simulink model "AMR_ManualModeController_23b"  (R2023b)
settings: Solver=FixedStepAuto  StartTime=0.0  StopTime=inf  FixedStep=1e-3  RelTol=1e-3
model workspace (MAT data in the model file):
  mdlWSDbList = "C:\Users\matlab.cut\Desktop\AMR\canbus_files\tramontina_database_mobotic.dbc"
  mobotic_mechanical_offset = -30
libraries: hdlsllib x4, speedgoatlib_IO60X_IO69X x3, tramontina_database_moboticlib x3, slrealtimeutilitieslib x1
settings Model: Creator=matlab.cut  LastModifiedBy=matlab.cut
settings SolverCC: ConcurrentTasks=on  PositivePriorityOrder=on  AutoInsertRateTranBlk=on
settings OptimizationCC: BlockReduction=off  OptimizeBlockIOStorage=off
settings DebuggingCC: TasksWithSamePriorityMsg=none
settings HardwareCC: ProdBitPerLong=64  ProdLongLongMode=on  ProdHWDeviceType=Intel->x86-64 (Linux 64)
settings ModelReferenceCC: ModelReferenceNumInstancesAllowed=Single
settings RTWCC: Description=Simulink Real-Time  SystemTargetFile=slrealtime.tlc  TemplateMakefile=slrealtime_default_tmf  Toolchain=Simulink Real-Time Toolchain  BuildConfiguration=Faster Runs  CodeExecutionProfiling=on  TargetLang=C++
settings CodeAppCC: MaxIdLength=127

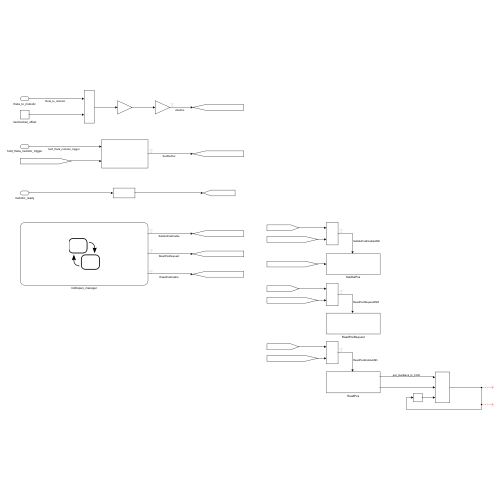
[thumbnail: Simulink's stored preview of the top-level diagram]
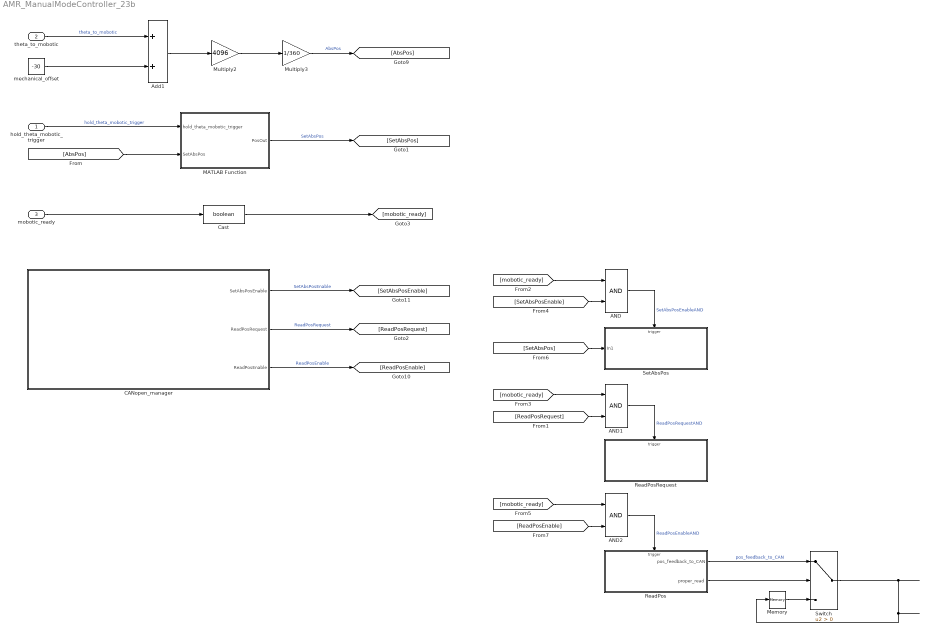
== system AMR_ManualModeController_23b ==
  hold_theta_mobotic_trigger : Inport  OutDataTypeStr=boolean
  theta_to_mobotic : Inport  Port=2
  mobotic_ready : Inport  Port=3  OutDataTypeStr=boolean
  AND : Logic  AllPortsSameDT=off  OutDataTypeStr=boolean
  AND1 : Logic  AllPortsSameDT=off  OutDataTypeStr=boolean
  AND2 : Logic  AllPortsSameDT=off  OutDataTypeStr=boolean
  Add1 : Sum
  CANopen_manager : Stateflow chart  TreatAsAtomicUnit=on
  Cast : DataTypeConversion  OutDataTypeStr=boolean  SaturateOnIntegerOverflow=off  RndMeth=Floor
  MATLAB Function : MATLAB Function  TreatAsAtomicUnit=on
  Memory : Memory
  Multiply2 : Gain  Gain=4096
  Multiply3 : Gain  Gain=1/360
  ReadPos : Subsystem  TreatAsAtomicUnit=on
  ReadPosRequest : Subsystem  TreatAsAtomicUnit=on
  SetAbsPos : Subsystem  TreatAsAtomicUnit=on
  Switch : Switch  Criteria=u2 > Threshold  SaturateOnIntegerOverflow=off  InputSameDT=off
  mechanical_offset : Constant  Value=-30
  wires:
  Multiply3/1 -> [AbsPos]  "AbsPos"
  CANopen_manager/3(ReadPosEnable) -> [ReadPosEnable]  "ReadPosEnable"
  mechanical_offset/1 -> Add1/2
  Add1/1 -> Multiply2/1
  [SetAbsPos] -> SetAbsPos/1(In1)
  Multiply2/1 -> Multiply3/1
  CANopen_manager/1(SetAbsPosEnable) -> [SetAbsPosEnable]  "SetAbsPosEnable"
  theta_to_mobotic/1 -> Add1/1  "theta_to_mobotic"
  [AbsPos] -> MATLAB Function/2(SetAbsPos)
  MATLAB Function/1(PosOut) -> [SetAbsPos]  "SetAbsPos"
  hold_theta_mobotic_trigger/1 -> MATLAB Function/1(hold_theta_mobotic_trigger)  "hold_theta_mobotic_trigger"
  CANopen_manager/2(ReadPosRequest) -> [ReadPosRequest]  "ReadPosRequest"
  ReadPos/2(proper_read) -> Switch/2
  Memory/1 -> Switch/3
  ReadPos/1(pos_feedback_to_CAN) -> Switch/1  "pos_feedback_to_CAN"
  Switch/1 -> Memory/1
  mobotic_ready/1 -> Cast/1
  AND/1 -> SetAbsPos/Trigger  "SetAbsPosEnableAND"
  [SetAbsPosEnable] -> AND/2
  [mobotic_ready] -> AND/1
  [mobotic_ready] -> AND1/1
  AND1/1 -> ReadPosRequest/Trigger  "ReadPosRequestAND"
  [ReadPosRequest] -> AND1/2
  [mobotic_ready] -> AND2/1
  [ReadPosEnable] -> AND2/2
  AND2/1 -> ReadPos/Trigger  "ReadPosEnableAND"
  Cast/1 -> [mobotic_ready]

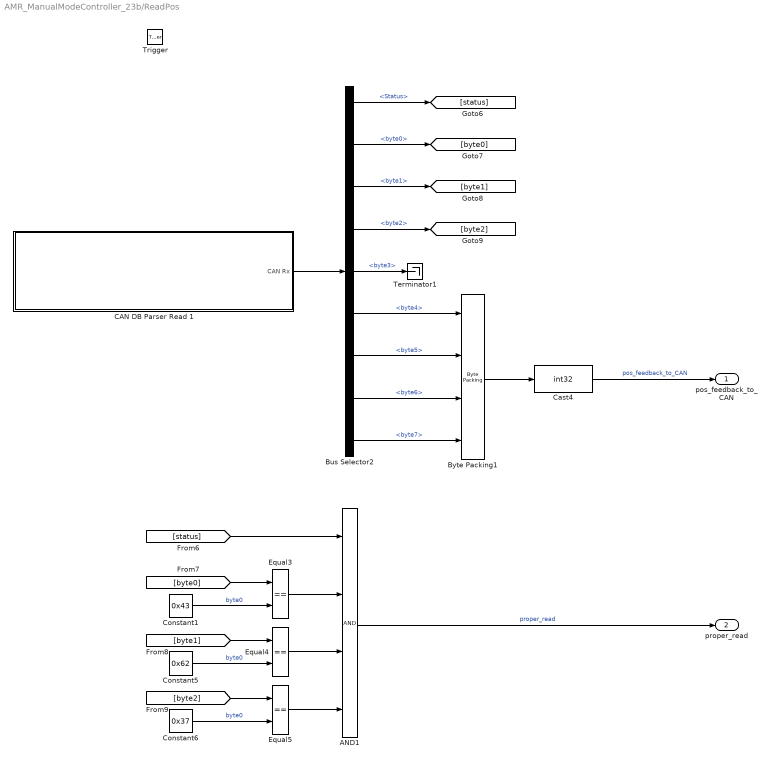
== system AMR_ManualModeController_23b/ReadPos ==
  Trigger : TriggerPort  VariantControl=(inherit)  PortDimensions=1
  AND1 : Logic  Inputs=4  AllPortsSameDT=off  OutDataTypeStr=boolean
  Bus Selector2 : BusSelector  OutputSignals=ID1459_feedback_word.MessageStatus.Status,ID1459_feedback_word.byte0,ID1459_feedback_word.byte1,ID1459_feedback_word.byte2,ID1459_feedback_word.byte3,ID1459_feedback_word.byte4,ID1459_feedback_word.byte5,ID1459_feedback_word.byte6,ID1459_feedback_word.byte7
  Byte Packing1 : slrealtimeutilitieslib/Byte Packing  MaskPackedDataType=int32  MaskUnpackedDataTypes={'uint8','uint8','uint8','uint8'}  MaskAlignment=1
  CAN DB Parser Read 1 : Subsystem
      settings: OpenFcn=sg_can.OpenFcnRead;
      mask Help: eval('sg.utils.help.show(''io_main/refentry_ref_can_ofa_parsing_read'');')
      mask Display: disp('Speedgoat\nIO691\nCAN DB Parser Read\nModule ID: IO691 - Module ID 1\nChannel:  1\ntramontina_database_mobotic.dbc ');
  Cast4 : DataTypeConversion  OutDataTypeStr=int32  SaturateOnIntegerOverflow=off  RndMeth=Floor
  Constant1 : Constant  Value=0x43
  Constant5 : Constant  Value=0x62
  Constant6 : Constant  Value=0x37
  Equal3 : RelationalOperator  Operator===  OutDataTypeStr=boolean  RndMeth=Simplest  InputSameDT=off
  Equal4 : RelationalOperator  Operator===  OutDataTypeStr=boolean  RndMeth=Simplest  InputSameDT=off
  Equal5 : RelationalOperator  Operator===  OutDataTypeStr=boolean  RndMeth=Simplest  InputSameDT=off
  Terminator1 : Terminator
  pos_feedback_to_CAN : Outport
  proper_read : Outport  Port=2
  wires:
  Equal5/1 -> AND1/4
  [byte0] -> Equal3/1
  Constant5/1 -> Equal4/2  "byte0"
  Bus Selector2/5 -> Terminator1/1  "<byte3>"
  [byte1] -> Equal4/1
  [byte2] -> Equal5/1
  Bus Selector2/9 -> Byte Packing1/4  "<byte7>"
  Bus Selector2/4 -> [byte2]  "<byte2>"
  [status] -> AND1/1
  Bus Selector2/2 -> [byte0]  "<byte0>"
  Bus Selector2/1 -> [status]  "<Status>"
  Bus Selector2/8 -> Byte Packing1/3  "<byte6>"
  Equal4/1 -> AND1/3
  AND1/1 -> proper_read/1  "proper_read"
  Bus Selector2/7 -> Byte Packing1/2  "<byte5>"
  Equal3/1 -> AND1/2
  Byte Packing1/1 -> Cast4/1
  CAN DB Parser Read 1/1(CAN Rx) -> Bus Selector2/1
  Bus Selector2/6 -> Byte Packing1/1  "<byte4>"
  Constant6/1 -> Equal5/2  "byte0"
  Bus Selector2/3 -> [byte1]  "<byte1>"
  Constant1/1 -> Equal3/2  "byte0"
  Cast4/1 -> pos_feedback_to_CAN/1  "pos_feedback_to_CAN"

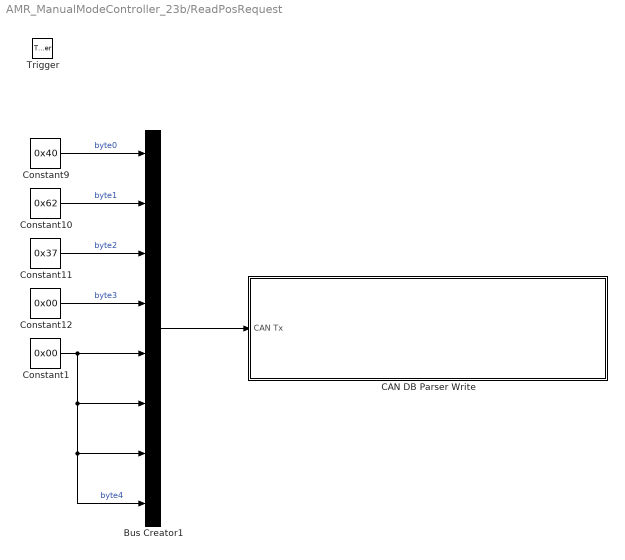
== system AMR_ManualModeController_23b/ReadPosRequest ==
  Trigger : TriggerPort  VariantControl=(inherit)  PortDimensions=1
  Bus Creator1 : BusCreator  Inputs=8
  "CAN DB Parser Write " : Subsystem
      settings: OpenFcn=sg_can.OpenFcnWrite;
      mask Help: eval('sg.utils.help.show(''io_main/refentry_ref_can_ofa_parsing_write'');')
      mask Display: disp('Speedgoat\nIO691\nCAN DB Parser Write\nModule ID: IO691 - Module ID 1\nChannel:  1\ntramontina_database_mobotic.dbc ');
  Constant1 : Constant  Value=0x00
  Constant10 : Constant  Value=0x62
  Constant11 : Constant  Value=0x37
  Constant12 : Constant  Value=0x00
  Constant9 : Constant  Value=0x40
  wires:
  Constant12/1 -> Bus Creator1/4  "byte3"
  Bus Creator1/1 -> "CAN DB Parser Write "/1(CAN Tx)
  Constant1/1 -> Bus Creator1/8, Bus Creator1/7, Bus Creator1/6, Bus Creator1/5  "byte4"
  Constant10/1 -> Bus Creator1/2  "byte1"
  Constant11/1 -> Bus Creator1/3  "byte2"
  Constant9/1 -> Bus Creator1/1  "byte0"

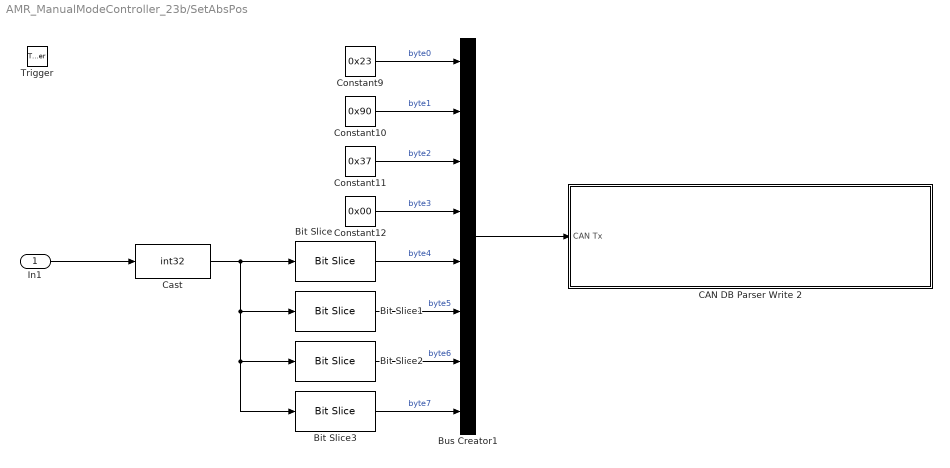
== system AMR_ManualModeController_23b/SetAbsPos ==
  In1 : Inport
  Trigger : TriggerPort  VariantControl=(inherit)  PortDimensions=1
  Bit Slice : hdlsllib/Logic and Bit Operations/Bit Slice  lidx=7  ridx=0
  Bit Slice1 : hdlsllib/Logic and Bit Operations/Bit Slice  lidx=15  ridx=8
  Bit Slice2 : hdlsllib/Logic and Bit Operations/Bit Slice  lidx=23  ridx=16
  Bit Slice3 : hdlsllib/Logic and Bit Operations/Bit Slice  lidx=31  ridx=24
  Bus Creator1 : BusCreator  Inputs=8
  CAN DB Parser Write 2 : Subsystem
      settings: OpenFcn=sg_can.OpenFcnWrite;
      mask Help: eval('sg.utils.help.show(''io_main/refentry_ref_can_ofa_parsing_write'');')
      mask Display: disp('Speedgoat\nIO691\nCAN DB Parser Write\nModule ID: IO691 - Module ID 1\nChannel:  1\ntramontina_database_mobotic.dbc ');
  Cast : DataTypeConversion  OutDataTypeStr=int32  SaturateOnIntegerOverflow=off  RndMeth=Floor
  Constant10 : Constant  Value=0x90
  Constant11 : Constant  Value=0x37
  Constant12 : Constant  Value=0x00
  Constant9 : Constant  Value=0x23
  wires:
  Constant9/1 -> Bus Creator1/1  "byte0"
  Constant12/1 -> Bus Creator1/4  "byte3"
  Constant11/1 -> Bus Creator1/3  "byte2"
  Bus Creator1/1 -> CAN DB Parser Write 2/1(CAN Tx)
  Constant10/1 -> Bus Creator1/2  "byte1"
  Bit Slice/1 -> Bus Creator1/5  "byte4"
  Bit Slice1/1 -> Bus Creator1/6  "byte5"
  Bit Slice2/1 -> Bus Creator1/7  "byte6"
  Bit Slice3/1 -> Bus Creator1/8  "byte7"
  In1/1 -> Cast/1
  Cast/1 -> Bit Slice3/1, Bit Slice2/1, Bit Slice1/1, Bit Slice/1

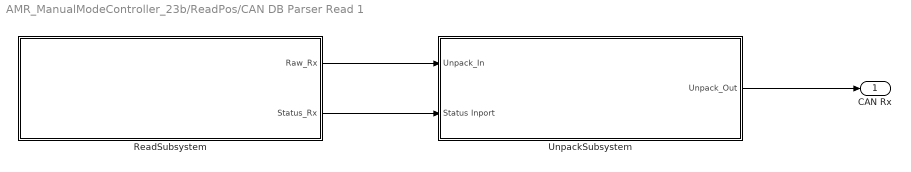
== system AMR_ManualModeController_23b/ReadPos/CAN DB Parser Read 1 ==
  ReadSubsystem : Subsystem
  UnpackSubsystem : Subsystem
  CAN Rx : Outport
  wires:
  ReadSubsystem/1(Raw_Rx) -> UnpackSubsystem/1(Unpack_In)
  ReadSubsystem/2(Status_Rx) -> UnpackSubsystem/2(Status Inport)
  UnpackSubsystem/1(Unpack_Out) -> CAN Rx/1

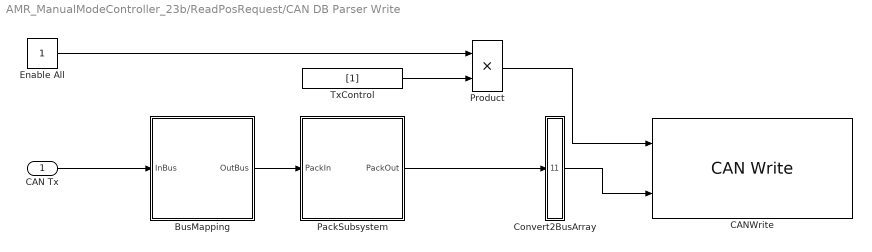
== system AMR_ManualModeController_23b/ReadPosRequest/CAN DB Parser Write  ==
  CAN Tx : Inport
  BusMapping : Subsystem
  CANWrite : speedgoatlib_IO60X_IO69X/CAN/CAN Write   moduleType=IO691  id=1  channel=1  canType=CAN (HS)  messageType=CAN (HS)  useBusIn=on  numOfMsg=1  enableInput=on  enableStatusPort=off  ts=-1  initValues=[691 1 -1 0 1 1 0 1 1 1]
  Convert2BusArray : Subsystem
  Enable All : Constant  OutDataTypeStr=boolean
  PackSubsystem : Subsystem
  Product : Product  OutDataTypeStr=uint32
  TxControl : Constant  Value=[1]  OutDataTypeStr=uint32
  wires:
  PackSubsystem/1(PackOut) -> Convert2BusArray/1(InBus)
  Convert2BusArray/1(BusArrayOut) -> CANWrite/2
  Product/1 -> CANWrite/1
  TxControl/1 -> Product/2
  Enable All/1 -> Product/1
  CAN Tx/1 -> BusMapping/1(InBus)
  BusMapping/1(OutBus) -> PackSubsystem/1(PackIn)

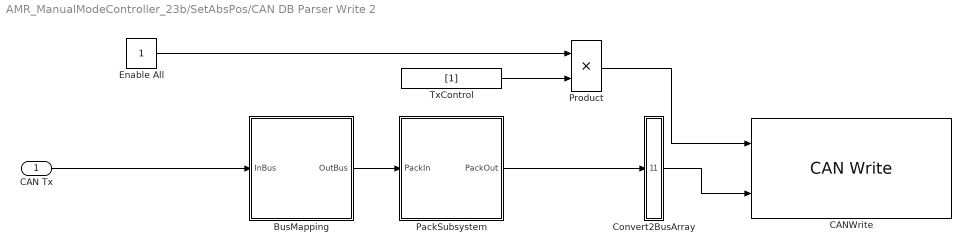
== system AMR_ManualModeController_23b/SetAbsPos/CAN DB Parser Write 2 ==
  CAN Tx : Inport
  BusMapping : Subsystem
  CANWrite : speedgoatlib_IO60X_IO69X/CAN/CAN Write   moduleType=IO691  id=1  channel=1  canType=CAN (HS)  messageType=CAN (HS)  useBusIn=on  numOfMsg=1  enableInput=on  enableStatusPort=off  ts=-1  initValues=[691 1 -1 0 1 1 0 1 1 1]
  Convert2BusArray : Subsystem
  Enable All : Constant  OutDataTypeStr=boolean
  PackSubsystem : Subsystem
  Product : Product  OutDataTypeStr=uint32
  TxControl : Constant  Value=[1]  OutDataTypeStr=uint32
  wires:
  PackSubsystem/1(PackOut) -> Convert2BusArray/1(InBus)
  Convert2BusArray/1(BusArrayOut) -> CANWrite/2
  Product/1 -> CANWrite/1
  TxControl/1 -> Product/2
  Enable All/1 -> Product/1
  CAN Tx/1 -> BusMapping/1(InBus)
  BusMapping/1(OutBus) -> PackSubsystem/1(PackIn)

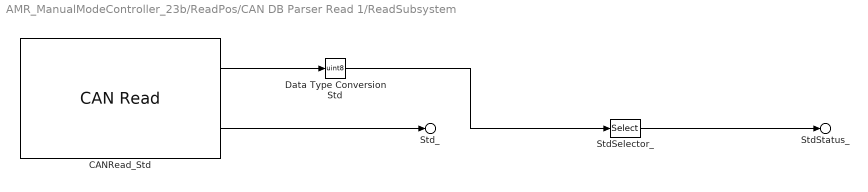
== system AMR_ManualModeController_23b/ReadPos/CAN DB Parser Read 1/ReadSubsystem ==
  CANRead_Std : speedgoatlib_IO60X_IO69X/CAN/CAN Read   moduleType=IO691  id=1  channel=1  canType=CAN (HS)  messageType=CAN (HS)  useBusOut=on  HasMulRead=Specify by IDs  MsgIDlist=[1459]  isEFF=off  LabelInHex=off  enableInput=off  initValues=[691 1 -1 0 1 1 0 1 2 0 1 1459]  ts=-1
  Data Type ConversionStd : DataTypeConversion  OutDataTypeStr=uint8  SaturateOnIntegerOverflow=off  RndMeth=Floor
  StdSelector_ : Selector  IndexOptions=Index vector (dialog)  Indices=1  OutputSizes=1
  Std_ : Outport  PortName=Raw_Rx  Element=Std.ID1459
  StdStatus_ : Outport  Port=2  PortName=Status_Rx  Element=Std.ID1459
  wires:
  CANRead_Std/1 -> Data Type ConversionStd/1
  CANRead_Std/2 -> Std_/1
  Data Type ConversionStd/1 -> StdSelector_/1
  StdSelector_/1 -> StdStatus_/1

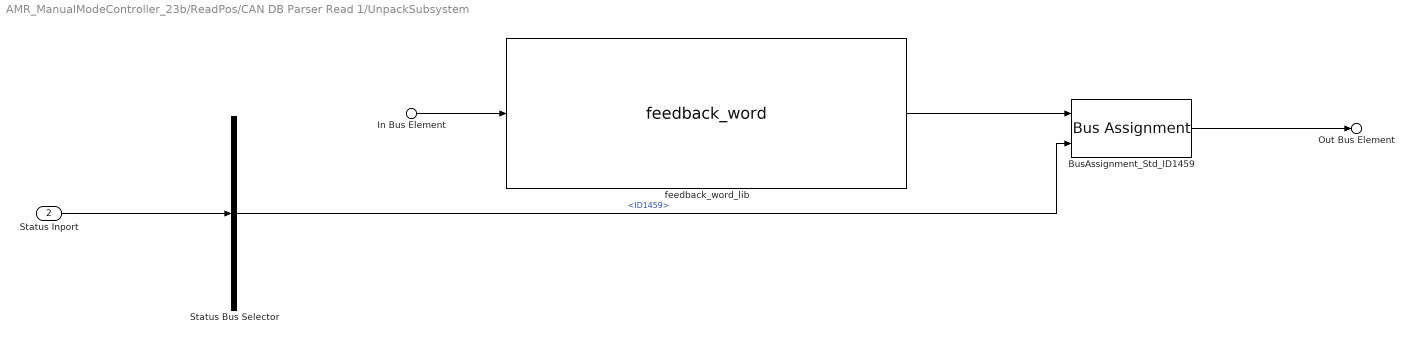
== system AMR_ManualModeController_23b/ReadPos/CAN DB Parser Read 1/UnpackSubsystem ==
  In Bus Element : Inport  PortName=Unpack_In  Element=Std.ID1459
  Status Inport : Inport  Port=2
  BusAssignment_Std_ID1459 : BusAssignment  AssignedSignals=MessageStatus.Status
  Status Bus Selector : BusSelector  OutputSignals=Std.ID1459
  feedback_word_lib : tramontina_database_moboticlib/CAN unpack/feedback_word  SystemSampleTime=-1  VariantActivationTime=update diagram  AllowFlexibleInterface=on  Latency=0  AutoFrameSizeCalculation=off
  Out Bus Element : Outport  PortName=Unpack_Out  Element=ID1459_feedback_word
  wires:
  In Bus Element/1 -> feedback_word_lib/1
  feedback_word_lib/1 -> BusAssignment_Std_ID1459/1
  BusAssignment_Std_ID1459/1 -> Out Bus Element/1
  Status Inport/1 -> Status Bus Selector/1
  Status Bus Selector/1 -> BusAssignment_Std_ID1459/2  "<ID1459>"

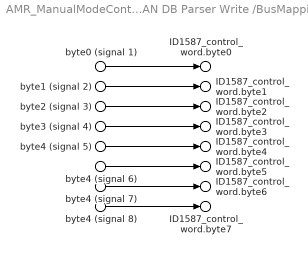
== system AMR_ManualModeController_23b/ReadPosRequest/CAN DB Parser Write /BusMapping ==
  byte0 (signal 1) : Inport  PortName=InBus  Element=byte0 (signal 1)
  byte1 (signal 2) : Inport  PortName=InBus  Element=byte1 (signal 2)
  byte2 (signal 3) : Inport  PortName=InBus  Element=byte2 (signal 3)
  byte3 (signal 4) : Inport  PortName=InBus  Element=byte3 (signal 4)
  byte4 (signal 5) : Inport  PortName=InBus  Element=byte4 (signal 5)
  byte4 (signal 6) : Inport  PortName=InBus  Element=byte4 (signal 6)
  byte4 (signal 7) : Inport  PortName=InBus  Element=byte4 (signal 7)
  byte4 (signal 8) : Inport  PortName=InBus  Element=byte4 (signal 8)
  ID1587_control_word.byte0 : Outport  PortName=OutBus  Element=ID1587_control_word.byte0
  ID1587_control_word.byte1 : Outport  PortName=OutBus  Element=ID1587_control_word.byte1
  ID1587_control_word.byte2 : Outport  PortName=OutBus  Element=ID1587_control_word.byte2
  ID1587_control_word.byte3 : Outport  PortName=OutBus  Element=ID1587_control_word.byte3
  ID1587_control_word.byte4 : Outport  PortName=OutBus  Element=ID1587_control_word.byte4
  ID1587_control_word.byte5 : Outport  PortName=OutBus  Element=ID1587_control_word.byte5
  ID1587_control_word.byte6 : Outport  PortName=OutBus  Element=ID1587_control_word.byte6
  ID1587_control_word.byte7 : Outport  PortName=OutBus  Element=ID1587_control_word.byte7
  wires:
  byte0 (signal 1)/1 -> ID1587_control_word.byte0/1
  byte1 (signal 2)/1 -> ID1587_control_word.byte1/1
  byte2 (signal 3)/1 -> ID1587_control_word.byte2/1
  byte3 (signal 4)/1 -> ID1587_control_word.byte3/1
  byte4 (signal 5)/1 -> ID1587_control_word.byte4/1
  byte4 (signal 6)/1 -> ID1587_control_word.byte5/1
  byte4 (signal 7)/1 -> ID1587_control_word.byte6/1
  byte4 (signal 8)/1 -> ID1587_control_word.byte7/1

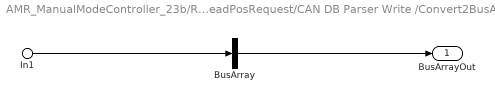
== system AMR_ManualModeController_23b/ReadPosRequest/CAN DB Parser Write /Convert2BusArray ==
  In1 : Inport  PortName=InBus  Element=ID1587_control_word
  BusArray : Concatenate  NumInputs=1
  BusArrayOut : Outport
  wires:
  In1/1 -> BusArray/1
  BusArray/1 -> BusArrayOut/1

== system AMR_ManualModeController_23b/ReadPosRequest/CAN DB Parser Write /PackSubsystem ==
  In Bus Element : Inport  PortName=PackIn  Element=ID1587_control_word
  control_word_lib : tramontina_database_moboticlib/CAN pack/control_word  SystemSampleTime=-1  VariantActivationTime=update diagram  AllowFlexibleInterface=on  Latency=0  AutoFrameSizeCalculation=off
  In Bus Element1 : Outport  PortName=PackOut  Element=ID1587_control_word
  wires:
  In Bus Element/1 -> control_word_lib/1
  control_word_lib/1 -> In Bus Element1/1

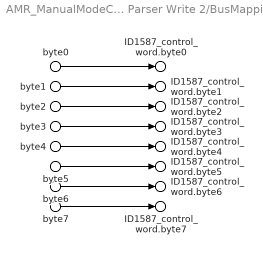
== system AMR_ManualModeController_23b/SetAbsPos/CAN DB Parser Write 2/BusMapping ==
  byte0 : Inport  PortName=InBus  Element=byte0
  byte1 : Inport  PortName=InBus  Element=byte1
  byte2 : Inport  PortName=InBus  Element=byte2
  byte3 : Inport  PortName=InBus  Element=byte3
  byte4 : Inport  PortName=InBus  Element=byte4
  byte5 : Inport  PortName=InBus  Element=byte5
  byte6 : Inport  PortName=InBus  Element=byte6
  byte7 : Inport  PortName=InBus  Element=byte7
  ID1587_control_word.byte0 : Outport  PortName=OutBus  Element=ID1587_control_word.byte0
  ID1587_control_word.byte1 : Outport  PortName=OutBus  Element=ID1587_control_word.byte1
  ID1587_control_word.byte2 : Outport  PortName=OutBus  Element=ID1587_control_word.byte2
  ID1587_control_word.byte3 : Outport  PortName=OutBus  Element=ID1587_control_word.byte3
  ID1587_control_word.byte4 : Outport  PortName=OutBus  Element=ID1587_control_word.byte4
  ID1587_control_word.byte5 : Outport  PortName=OutBus  Element=ID1587_control_word.byte5
  ID1587_control_word.byte6 : Outport  PortName=OutBus  Element=ID1587_control_word.byte6
  ID1587_control_word.byte7 : Outport  PortName=OutBus  Element=ID1587_control_word.byte7
  wires:
  byte0/1 -> ID1587_control_word.byte0/1
  byte1/1 -> ID1587_control_word.byte1/1
  byte2/1 -> ID1587_control_word.byte2/1
  byte3/1 -> ID1587_control_word.byte3/1
  byte4/1 -> ID1587_control_word.byte4/1
  byte5/1 -> ID1587_control_word.byte5/1
  byte6/1 -> ID1587_control_word.byte6/1
  byte7/1 -> ID1587_control_word.byte7/1

== system AMR_ManualModeController_23b/SetAbsPos/CAN DB Parser Write 2/Convert2BusArray ==
  In1 : Inport  PortName=InBus  Element=ID1587_control_word
  BusArray : Concatenate  NumInputs=1
  BusArrayOut : Outport
  wires:
  In1/1 -> BusArray/1
  BusArray/1 -> BusArrayOut/1

== system AMR_ManualModeController_23b/SetAbsPos/CAN DB Parser Write 2/PackSubsystem ==
  In Bus Element : Inport  PortName=PackIn  Element=ID1587_control_word
  control_word_lib : tramontina_database_moboticlib/CAN pack/control_word  SystemSampleTime=-1  VariantActivationTime=update diagram  AllowFlexibleInterface=on  Latency=0  AutoFrameSizeCalculation=off
  In Bus Element1 : Outport  PortName=PackOut  Element=ID1587_control_word
  wires:
  In Bus Element/1 -> control_word_lib/1
  control_word_lib/1 -> In Bus Element1/1

== matlab function AMR_ManualModeController_23b/MATLAB Function ==
  data: hold_theta_mobotic_trigger input; SetAbsPos input; PosOut output
function PosOut = fcn(hold_theta_mobotic_trigger, SetAbsPos)
% Function to select output depending on hold_theta_mobotic On/Off status

persistent PosAux  % Declaring PosAux as persistent to retain its value between function calls

if isempty(PosAux)  % Initialize PosAux if it's empty
    PosAux = 0;
end

if hold_theta_mobotic_trigger == 1
    PosOut = SetAbsPos;
    PosAux = PosOut;
else
    PosOut = PosAux;
end

== stateflow chart AMR_ManualModeController_23b/CANopen_manager ==
  state SetAbsPos
    % set flag to run SetAbsPos_Subsystem
    entry:
    SetAbsPosEnable = 1;
    ReadPosRequest = 0;
    ReadPosEnable = 0;
    exit:
    SetAbsPosEnable = 0;
    state=1;
  state ReadPosRequest
    entry:
    SetAbsPosEnable = 0;
    ReadPosRequest = 1;
    ReadPosEnable = 0;
    exit:
    ReadPosRequest=0;
    state=2;
  state ReadPosFeedback
    entry:
    SetAbsPosEnable = 0;
    ReadPosRequest = 0;
    ReadPosEnable = 1;
    exit:
    ReadPosEnable=0;
    state=3;
  (default) -> SetAbsPos : {SetAbsPosEnable=0}
  SetAbsPos -> ReadPosRequest : after(10,msec)
  (junction 29) -> SetAbsPos
  ReadPosRequest -> ReadPosFeedback : after(5,msec)
  ReadPosFeedback -> (junction 29) : after(5,msec)
  data: SetAbsPosEnable output; ReadPosRequest output; ReadPosEnable output; state local
